simulink model "TireForces"  (R2019a)
settings: Solver=ode15s  StartTime=0.0  StopTime=10  RelTol=1e-3
values from neighbouring files (symbols this model uses):
  Bx = 10    [AuE881_HW5_Zhai_Kexuan_HW5_initialization.m]
  By = 12.5    [AuE881_HW5_Zhai_Kexuan_HW5_initialization.m]
  Bz = 20    [AuE881_HW5_Zhai_Kexuan_HW5_initialization.m]
  Cx = 1.9    [AuE881_HW5_Zhai_Kexuan_HW5_initialization.m]
  Cy = 1.2    [AuE881_HW5_Zhai_Kexuan_HW5_initialization.m]
  Cz = 2.4    [AuE881_HW5_Zhai_Kexuan_HW5_initialization.m]
  Dx = 1    [AuE881_HW5_Zhai_Kexuan_HW5_initialization.m]
  Dy = -1    [AuE881_HW5_Zhai_Kexuan_HW5_initialization.m]
  Dz = 0.011    [AuE881_HW5_Zhai_Kexuan_HW5_initialization.m]
  Ex = 0.8    [AuE881_HW5_Zhai_Kexuan_HW5_initialization.m]
  Ey = -1    [AuE881_HW5_Zhai_Kexuan_HW5_initialization.m]
  Ez = -1    [AuE881_HW5_Zhai_Kexuan_HW5_initialization.m]
settings Model: Creator=paredis  LastModifiedBy=paredis
settings DataIOCC: SaveOutput=off  SaveTime=off

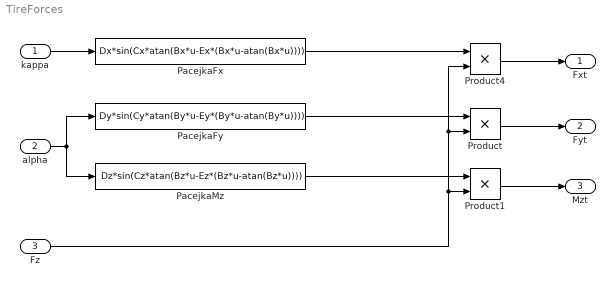
== system TireForces ==
  kappa : Inport  OutDataTypeStr=double  PortDimensions=1  SampleTime=0
  alpha : Inport  Port=2  OutDataTypeStr=double  PortDimensions=1  SampleTime=0
  Fz : Inport  Port=3  OutDataTypeStr=double  PortDimensions=1
  PacejkaFx : Fcn  Expr=Dx*sin(Cx*atan(Bx*u-Ex*(Bx*u-atan(Bx*u))))
  PacejkaFy : Fcn  Expr=Dy*sin(Cy*atan(By*u-Ey*(By*u-atan(By*u))))
  PacejkaMz : Fcn  Expr=Dz*sin(Cz*atan(Bz*u-Ez*(Bz*u-atan(Bz*u))))
  Product : Product
  Product1 : Product
  Product4 : Product
  Fxt : Outport  OutDataTypeStr=double  PortDimensions=1  SampleTime=0
  Fyt : Outport  Port=2  OutDataTypeStr=double  PortDimensions=1  SampleTime=0
  Mzt : Outport  Port=3  OutDataTypeStr=double  PortDimensions=1  SampleTime=0
  wires:
  kappa/1 -> PacejkaFx/1
  alpha/1 -> PacejkaMz/1, PacejkaFy/1
  PacejkaFy/1 -> Product/1
  Fz/1 -> Product1/2, Product/2, Product4/2
  PacejkaFx/1 -> Product4/1
  Product4/1 -> Fxt/1
  Product/1 -> Fyt/1
  Product1/1 -> Mzt/1
  PacejkaMz/1 -> Product1/1
